simulink model "experimental_setup"  (R2013b)
settings: Solver=ode45  StartTime=0.0  StopTime=0.05  FixedStep=0.00001  RelTol=1e-4
InitFcn:
  | init_experimental_setup
values from neighbouring files (symbols this model uses):
  aif_cal = transferMatrix    [init_experimental_setup.m]    (also in inspect_simulinkAIF.m = (cm.'*cm)\cm.')
  K1d = c2d( K1, Ts/2)    [init_experimental_setup.m]
  sampleTimeWavefrontSensor = Ts    (= 0.00125)    [init_experimental_setup.m]
undefined symbols (not defined in the file): delayWavefront, dimSlopeMatrix, dimSquareMatrix
libraries: LibraryExperimental x8
settings Model: Creator=steffen  LastModifiedBy=smauch
settings SolverCC: AutoInsertRateTranBlk=on
settings DataIOCC: SignalLoggingSaveFormat=ModelDataLogs  ReturnWorkspaceOutputs=on
settings OptimizationCC: ExpressionDepthLimit=2147483647
settings DebuggingCC: StateNameClashWarn=warning
settings HardwareCC: ProdHWDeviceType=Generic->Unspecified (assume 32-bit Generic)
settings GRTTargetCC: CombineOutputUpdateFcns=off  GRTInterface=on

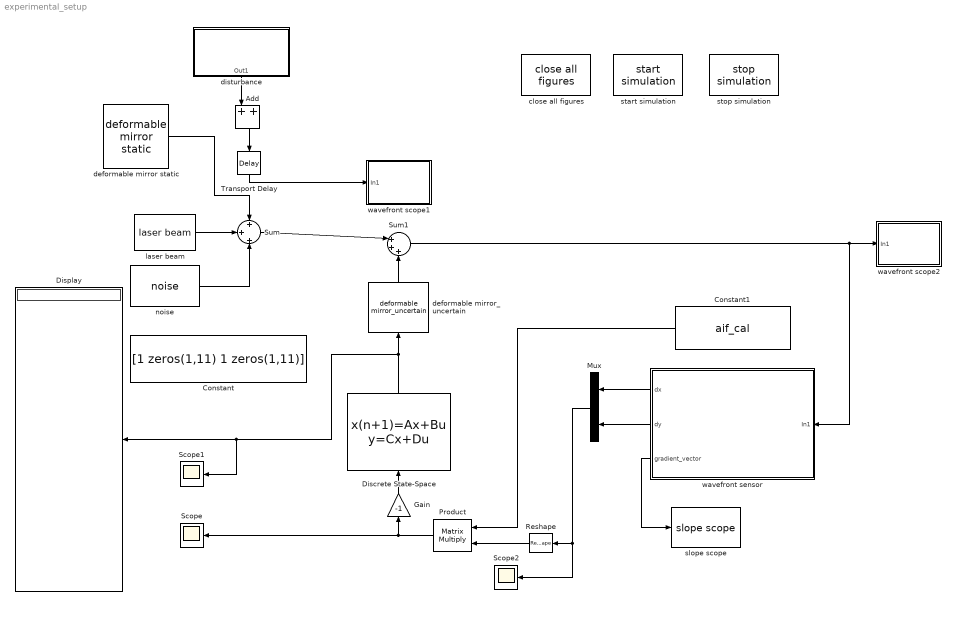
== system experimental_setup ==
  Add : Sum
  Constant : Constant  Value=[1 zeros(1,11) 1 zeros(1,11)]
  Constant1 : Constant  Value=aif_cal  VectorParams1D=off
  Discrete State-Space : DiscreteStateSpace  A=K1d.A  B=K1d.B  C=K1d.C  D=K1d.D  SampleTime=sampleTimeWavefrontSensor
  Display : Display
  Gain : Gain  Gain=-1
  Mux : Mux  Inputs=2
  Product : Product  Multiplication=Matrix(*)
  Reshape : Reshape  OutputDimensionality=Column vector (2-D)
  Scope : Scope
      settings: TimeRange=0.025  YMin=-0.4  YMax=1.2
  Scope1 : Scope
      settings: YMin=-2.5e+06  YMax=6e+06
  Scope2 : Scope
      settings: YMin=-0.45  YMax=0.4  SaveName=ScopeData2
  Sum : Sum  Inputs=+|+|+
  Sum1 : Sum  Inputs=|+++
  Transport Delay : TransportDelay  DelayTime=0.1
  close all figures : LibraryExperimental/close all figures  SystemSampleTime=-1
  deformable mirror static : LibraryExperimental/deformable mirror static  dimActuator=dimActuator  dimMatrix=dimSquareMatrix  layoutActuator=layoutActuator  dm_static=DMmodel_static  input=staticDMInput  delay=0.0099
  deformable mirror_uncertain : LibraryExperimental/deformable mirror_uncertain  dimActuator=dimActuator  dimMatrix=dimSquareMatrix  layoutActuator=layoutActuator  model=DMmodel  uncertainty=0
  disturbance : Subsystem  mask{dimMatrix=dimSquareMatrix, zernik1=1, zernik2=-1, scale=5, rotate=45}
      mask prompts: dimMatrix "dimSquareMatrix"; zernik1 "Zernike1"; zernik2 "Zernike2"; rotate "rotate in deg"
      mask Display:
      | port_label('output', 1, 'y')
      | 
      | patch([0 0.5 1], [0 1 0],[0.7 0.6 0])
      | patch( [0.15 0.85 0.85 0.15], [0.6 0.6 0.4 0.4], [0.9 0.9 0.9] )
      | fprintf('stationar Zernike')
  laser beam : LibraryExperimental/laser beam  dimSquare=dimSquareMatrix
  noise : LibraryExperimental/noise  enable=on  dimSquare=dimSquareMatrix  Ts=sampleTimeWavefrontSensor  scaleNoise=25
  slope scope : LibraryExperimental/slope scope  sampleTime=0.1  dimMatrix=dimSlopeMatrix  enable=off  title='wavefront sensor'
  start simulation : LibraryExperimental/start simulation  SystemSampleTime=-1
  stop simulation : LibraryExperimental/stop simulation  SystemSampleTime=-1
  wavefront scope1 : Subsystem  mask{sampleTime=0.1, dimMatrix=dimSquareMatrix, enable=off, title='disturbance'}
      mask prompts: sampleTime "Sample Time"; dimMatrix "dimSquareMatrix"; enable "enable Scope"
      mask Display:
      | patch([0 0.5 1], [0 1 0],[1 0 0])
      | patch( [0.15 0.85 0.85 0.15], [0.6 0.6 0.4 0.4], [0.9 0.9 0.9] )
      | fprintf('Scope surf')
  wavefront scope2 : Subsystem  mask{sampleTime=0.05, dimMatrix=dimSquareMatrix, enable=on, title='laser beam'}
      mask prompts: sampleTime "Sample Time"; dimMatrix "dimSquareMatrix"; enable "enable Scope"
      mask Display:
      | patch([0 0.5 1], [0 1 0],[1 0 0])
      | patch( [0.15 0.85 0.85 0.15], [0.6 0.6 0.4 0.4], [0.9 0.9 0.9] )
      | fprintf('Scope surf')
  wavefront sensor : Subsystem  AncestorBlock=LibraryExperimental/wavefront sensor  mask{sampleTime=sampleTimeWavefrontSensor, dimMatrix_i=dimSquareMatrix, dimMatrix_o=dimSlopeMatrix, delay=delayWavefront, noiseSHWFS=0, scaleSHWFS=1/100, aperture=on}
      mask prompts: sampleTime "sample time of SHWFS"; dimMatrix_i "dimSquareMatrix Input"; dimMatrix_o "dimSquareMatrix Output"; delay "delay of SHWFS in ms"; noiseSHWFS "SHWFS noise"; scaleSHWFS "SHWFS scale"; aperture "enable circular aperture"
      mask Display:
      | image(imread('shacksensor.jpg'))
      | 
      | patch( [1 1 0.9 0.9],[0.4 0.6 0.6 0.4],[0.9 0.9 0.9] )
      | port_label('input', 1, 'u')
      | 
      | patch( [0 0 0.1 0.1],[0.9 0.75 0.75 0.9],[0.9 0.9 0.9] )
      | port_label('output', 1, 'dx')
      | 
      | patch( [0 0 0.1 0.1],[0.425 0.575 0.575 0.425],[0.9 0.9 0.9] )
      | port_label('output', 2, 'dy')
      | 
      | patch( [0 0 0.25 0.25],[0.1 0.25 0.25 0.1],[0.9 0.9 0.9] )
      | port_label('output', 3, 'wavefront')
  wires:
  laser beam/1 -> Sum/2
  noise/1 -> Sum/3
  Sum/1 -> Sum1/1
  wavefront sensor/3(gradient_vector) -> slope scope/1
  deformable mirror_uncertain/1 -> Sum1/3
  wavefront sensor/2(dy) -> Mux/2
  wavefront sensor/1(dx) -> Mux/1
  Transport Delay/1 -> wavefront scope1/1(In1)
  Sum1/1 -> wavefront sensor/1(In1), wavefront scope2/1(In1)
  Add/1 -> Transport Delay/1
  disturbance/1(Out1) -> Add/1
  Product/1 -> Gain/1, Scope/1
  Mux/1 -> Scope2/1, Reshape/1
  Reshape/1 -> Product/2
  Constant1/1 -> Product/1
  Gain/1 -> Discrete State-Space/1
  deformable mirror static/1 -> Sum/1
  Discrete State-Space/1 -> deformable mirror_uncertain/1, Scope1/1, Display/1

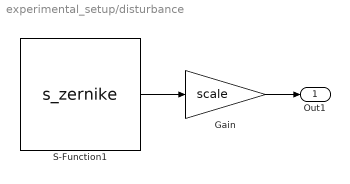
== system experimental_setup/disturbance ==
  Gain : Gain  Gain=scale
  S-Function1 : S-Function  FunctionName=s_zernike  Parameters=dimMatrix,zernik1,zernik2,rotate  EnableBusSupport=off
  Out1 : Outport
  wires:
  S-Function1/1 -> Gain/1
  Gain/1 -> Out1/1

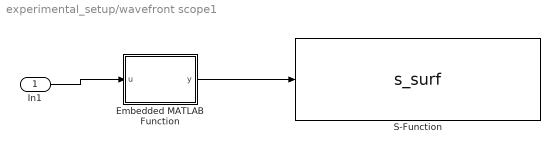
== system experimental_setup/wavefront scope1 ==
  In1 : Inport
  Embedded MATLAB Function : MATLAB Function  TreatAsAtomicUnit=on
  S-Function : S-Function  FunctionName=s_surf  Parameters=sampleTime,dimMatrix,enable,title  EnableBusSupport=off
  wires:
  In1/1 -> Embedded MATLAB Function/1(u)
  Embedded MATLAB Function/1(y) -> S-Function/1

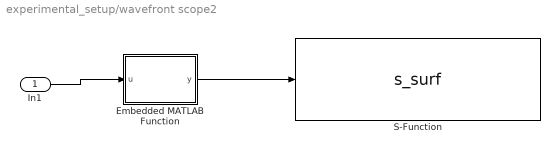
== system experimental_setup/wavefront scope2 ==
  In1 : Inport
  Embedded MATLAB Function : MATLAB Function  TreatAsAtomicUnit=on
  S-Function : S-Function  FunctionName=s_surf  Parameters=sampleTime,dimMatrix,enable,title  EnableBusSupport=off
  wires:
  Embedded MATLAB Function/1(y) -> S-Function/1
  In1/1 -> Embedded MATLAB Function/1(u)

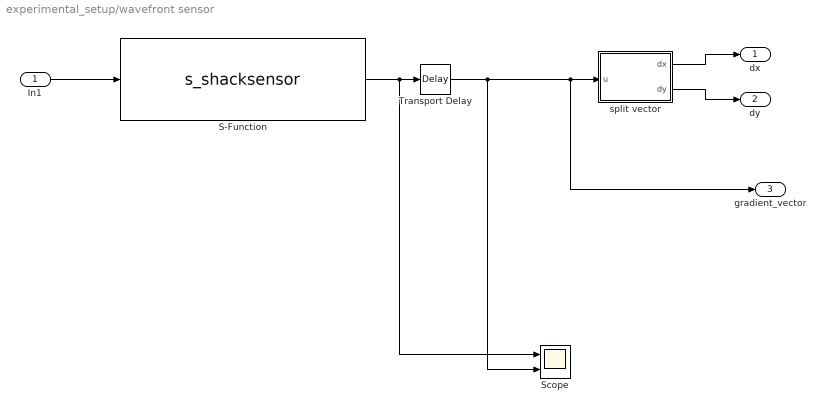
== system experimental_setup/wavefront sensor ==
  In1 : Inport
  S-Function : S-Function  FunctionName=s_shacksensor  Parameters=sampleTime,dimMatrix_i,dimMatrix_o,noiseSHWFS,scaleSHWFS,aperture  EnableBusSupport=off
  Scope : Scope  NumInputPorts=2
      settings: YMin=-5~-5  YMax=5~5  SaveName=ScopeData3
  Transport Delay : TransportDelay  DelayTime=delay*10^(-3)
  split vector : MATLAB Function  TreatAsAtomicUnit=on
  dx : Outport
  dy : Outport  Port=2
  gradient_vector : Outport  Port=3
  wires:
  Transport Delay/1 -> split vector/1(u), gradient_vector/1, Scope/2
  S-Function/1 -> Transport Delay/1, Scope/1
  In1/1 -> S-Function/1
  split vector/2(dy) -> dy/1
  split vector/1(dx) -> dx/1

== matlab function experimental_setup/wavefront scope2/Embedded MATLAB Function ==
  data: u input; y output
function y = fcn(u)
%#eml

y = u(:);

== matlab function experimental_setup/wavefront sensor/split vector ==
  data: dx output; u input; dy output
function [dx,dy] = fcn(u)
%#eml
u_length = length(u);

dx = u(1:u_length/2);
dy = u(u_length/2+1:u_length);

== matlab function experimental_setup/wavefront scope1/Embedded MATLAB Function ==
  data: u input; y output
function y = fcn(u)
%#eml

y = u(:);
